simulink model "Task1_sim"  (R2014a)
settings: Solver=ode45  StartTime=1  StopTime=2  RelTol=1e-3
settings Model: Creator=bunka  LastModifiedBy=bunka

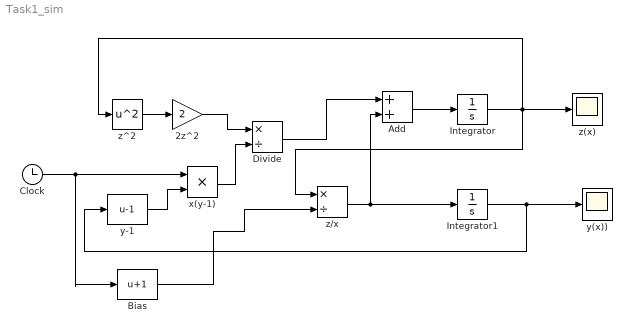
== system Task1_sim ==
  2z^2 : Gain  Gain=2
  Add : Sum
  Bias : Bias  Bias=1
  Clock : Clock
  Divide : Product  Inputs=*/
  Integrator : Integrator  InitialCondition=1/3
  Integrator1 : Integrator
  x(y-1) : Product
  y(x)) : Scope
  y-1 : Bias  Bias=-1
  z(x) : Scope
  z/x : Product  Inputs=*/
  z^2 : Math  Operator=square  SaturateOnIntegerOverflow=on
  wires:
  Integrator/1 -> z(x)/1, z^2/1, z/x/1
  Integrator1/1 -> y-1/1, y(x))/1
  z/x/1 -> Add/2, Integrator1/1
  Add/1 -> Integrator/1
  z^2/1 -> 2z^2/1
  x(y-1)/1 -> Divide/2
  2z^2/1 -> Divide/1
  Clock/1 -> Bias/1, x(y-1)/1
  y-1/1 -> x(y-1)/2
  Divide/1 -> Add/1
  Bias/1 -> z/x/2
